simulink model "Overforingsfunksjon_Rotasjon_samlet_PID"  (R2023b)
settings: Solver=VariableStepAuto  StartTime=0.0  StopTime=4  RelTol=1e-8
values from neighbouring files (symbols this model uses):
  D_phi = [M(4),rho_vann*Cd*A_phi*phi_2,(Zm*G-Zb*F_b)*cosd(thetha)*cosd(phi_1)]    [Overforingsfunksjon_Rotasjon.m]
  D_psi = [M(6),rho_vann*Cd*A_psi*psi_2]    [Overforingsfunksjon_Rotasjon.m]
  D_thetha = [M(5),rho_vann*Cd*A_thetha*thetha_2,(Zm*G-Zb*F_b)*cosd(thetha_1)]    [Overforingsfunksjon_Rotasjon.m]
settings Model: Creator=Anne Brit  LastModifiedBy=anneb
settings DataIOCC: InitialState=0.5

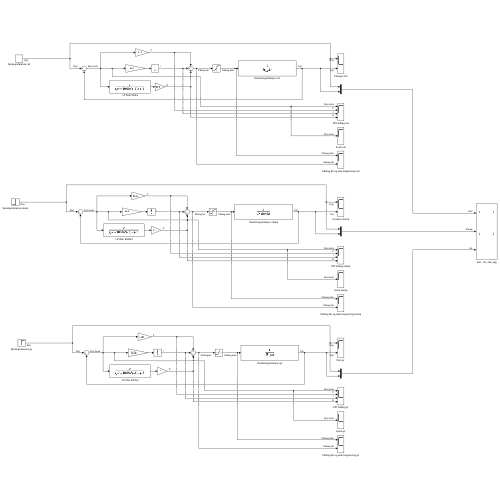
[thumbnail: Simulink's stored preview of the top-level diagram]
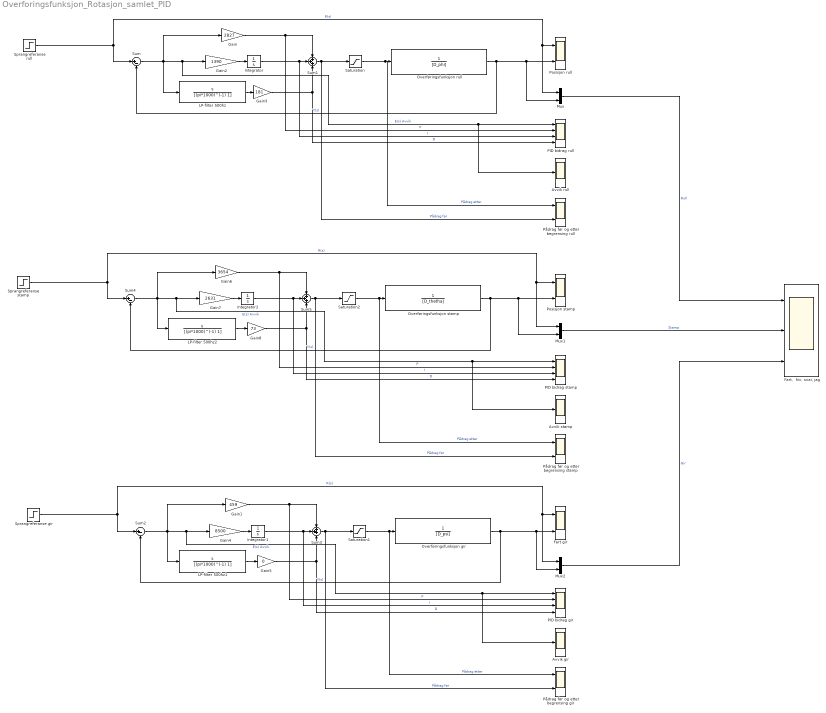
== system Overforingsfunksjon_Rotasjon_samlet_PID ==
  " LP-filter 500hz" : TransferFcn  Numerator=[1 0]  Denominator=[(pi*1000)^(-1) 1]
  " LP-filter 500hz1" : TransferFcn  Numerator=[1 0]  Denominator=[(pi*1000)^(-1) 1]
  " LP-filter 500hz2" : TransferFcn  Numerator=[1 0]  Denominator=[(pi*1000)^(-1) 1]
  Avvik gir : Scope
  Avvik rull : Scope
  Avvik stamp : Scope
  "Fart gir " : Scope  NumInputPorts=2
  "Fart,  hiv, svai, jag" : Scope  NumInputPorts=3
  Gain : Gain  Gain=2827
  Gain1 : Gain  Gain=459
  Gain2 : Gain  Gain=1390
  Gain3 : Gain  Gain=181
  Gain4 : Gain  Gain=8500
  Gain5 : Gain  Gain=0
  Gain6 : Gain  Gain=3654
  Gain7 : Gain  Gain=2631
  Gain8 : Gain  Gain=73
  Integrator : Integrator
  Integrator1 : Integrator
  Integrator2 : Integrator
  Mux : Mux  Inputs=2
  Mux1 : Mux  Inputs=2
  Mux2 : Mux  Inputs=2
  Overføringsfunksjon gir : TransferFcn  Denominator=[D_psi]
  "Overføringsfunksjon rull " : TransferFcn  Denominator=[D_phi]
  Overføringsfunksjon stamp : TransferFcn  Denominator=[D_thetha]
  PID bidrag gir : Scope  NumInputPorts=4
  PID bidrag rull : Scope  NumInputPorts=4
  PID bidrag stamp : Scope  NumInputPorts=4
  Posisjon rull : Scope  NumInputPorts=2
  Posisjon stamp : Scope  NumInputPorts=2
  Pådrag før og etter begrensing gir : Scope  NumInputPorts=2
  Pådrag før og etter begrensing rull : Scope  NumInputPorts=2
  Pådrag før og etter begrensing stamp : Scope  NumInputPorts=2
  Saturation : Saturate  UpperLimit=350  LowerLimit=-345
  Saturation1 : Saturate  UpperLimit=425  LowerLimit=-410
  Saturation2 : Saturate  UpperLimit=425  LowerLimit=-410
  Sprangreferanse gir : Step  After=0.39  SampleTime=0
  Sprangreferanse rull : Step  After=0.39  SampleTime=0
  Sprangreferanse stamp : Step  After=0.39  SampleTime=0
  Sum : Sum  Inputs=|+-
  Sum1 : Sum  Inputs=+++
  Sum2 : Sum  Inputs=|+-
  Sum3 : Sum  Inputs=+++
  Sum4 : Sum  Inputs=|+-
  Sum5 : Sum  Inputs=+++
  wires:
  "Overføringsfunksjon rull "/1 -> Sum/2, Mux/2, Posisjon rull/2  "Y(s)"
  Gain2/1 -> Integrator/1
  Sum/1 -> " LP-filter 500hz"/1, Gain/1, Gain2/1, PID bidrag rull/1, Avvik rull/1  "E(s) Avvik"
  Gain/1 -> Sum1/1, PID bidrag rull/2  "P"
  Gain3/1 -> Sum1/3, PID bidrag rull/4  "D"
  Sprangreferanse rull/1 -> Mux/1, Posisjon rull/1, Sum/1  "R(s)"
  Integrator/1 -> PID bidrag rull/3, Sum1/2  "I"
  Saturation/1 -> "Overføringsfunksjon rull "/1, Pådrag før og etter begrensing rull/1  "Pådrag etter"
  Sum1/1 -> Saturation/1, Pådrag før og etter begrensing rull/2  "Pådrag før"
  Sum3/1 -> Saturation1/1, Pådrag før og etter begrensing gir/2  "Pådrag før"
  Gain1/1 -> Sum3/1, PID bidrag gir/2  "P"
  Gain4/1 -> Integrator1/1
  Sprangreferanse gir/1 -> Mux2/1, "Fart gir "/1, Sum2/1  "R(s)"
  Integrator1/1 -> PID bidrag gir/3, Sum3/2  "I"
  " LP-filter 500hz1"/1 -> Gain5/1
  Gain5/1 -> Sum3/3, PID bidrag gir/4  "D"
  Sum2/1 -> " LP-filter 500hz1"/1, Gain1/1, Gain4/1, PID bidrag gir/1, Avvik gir/1  "E(s) Avvik"
  Overføringsfunksjon gir/1 -> Sum2/2, Mux2/2, "Fart gir "/2  "Y(s)"
  Saturation1/1 -> Pådrag før og etter begrensing gir/1, Overføringsfunksjon gir/1  "Pådrag etter"
  Overføringsfunksjon stamp/1 -> Sum4/2, Mux1/2, Posisjon stamp/2  "Y(s)"
  Sum4/1 -> " LP-filter 500hz2"/1, Gain6/1, Gain7/1, PID bidrag stamp/1, Avvik stamp/1  "E(s) Avvik"
  Sum5/1 -> Saturation2/1, Pådrag før og etter begrensing stamp/2  "Pådrag før"
  Gain6/1 -> Sum5/1, PID bidrag stamp/2  "P"
  Gain8/1 -> Sum5/3, PID bidrag stamp/4  "D"
  Saturation2/1 -> Pådrag før og etter begrensing stamp/1, Overføringsfunksjon stamp/1  "Pådrag etter"
  Integrator2/1 -> PID bidrag stamp/3, Sum5/2  "I"
  Gain7/1 -> Integrator2/1
  " LP-filter 500hz2"/1 -> Gain8/1
  Sprangreferanse stamp/1 -> Mux1/1, Posisjon stamp/1, Sum4/1  "R(s)"
  Mux1/1 -> "Fart,  hiv, svai, jag"/2  "Stamp"
  Mux/1 -> "Fart,  hiv, svai, jag"/1  "Rull"
  Mux2/1 -> "Fart,  hiv, svai, jag"/3  "Gir"
  " LP-filter 500hz"/1 -> Gain3/1
